simulink model "RobotArmControl"  (R2021a)
settings: Solver=FixedStepAuto  StartTime=0.0  StopTime=inf  RelTol=1e-3  EnableMultiTasking=on
InitFcn:
  | cBase=90;
  | cShoulder=90;
  | cElbow=90;
  | cWristVer=90;
  | cWristRot=90;
  | cGripper=73;
libraries: arduinolib x8
settings Model: SILPILModeSetting=veronly  ExtModeTrigDuration=2  Creator=loris  LastModifiedBy=angelo
settings OptimizationCC: EnhancedBackFolding=on  PassReuseOutputArgsAs=Individual arguments  ZeroExternalMemoryAtStartup=off  ZeroInternalMemoryAtStartup=off  MaxStackSize=64  OptimizeBlockOrder=speed  DifferentSizesBufferReuse=on  OptimizationCustomize=off  EfficientTunableParamExpr=on
settings DebuggingCC: ParameterTunabilityLossMsg=error
settings HardwareCC: ProdBitPerInt=16  ProdBitPerPointer=16  ProdBitPerSizeT=16  ProdBitPerPtrDiffT=16  ProdLargestAtomicFloat=None  ProdWordSize=8  ProdHWDeviceType=Atmel->AVR
settings SFSimCC: MATLABDynamicMemAlloc=off
settings RTWCC: SystemTargetFile=ert.tlc  HardwareBoard=Arduino Mega 2560  TemplateMakefile=ert_default_tmf  Toolchain=Arduino AVR  BuildConfiguration=Faster Runs
settings CodeAppCC: ForceParamTrailComments=on  IgnoreCustomStorageClasses=off  OperatorAnnotations=on  SimulinkDataObjDesc=on  SFDataObjDesc=on  InsertBlockDesc=on
settings ERTTargetCC: TargetLangStandard=C99 (ISO)  SupportContinuousTime=on  SupportVariableSizeSignals=on  ExtModeStaticAllocSize=2048  RootIOFormat=Structure reference

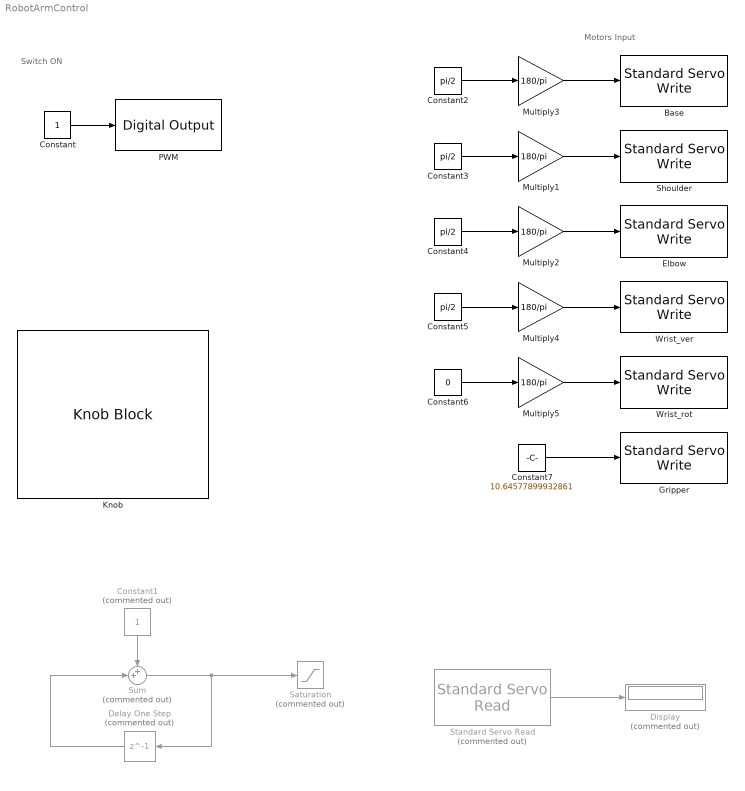
== system RobotArmControl ==
  note: Switch ON
  note: Motors Input
  Base : arduinolib/Standard Servo Write  pinNumber=11  ServoIndex=0  blockPlatform=ARDUINO
  Constant : Constant
  Constant1 : Constant  Commented=on
  Constant{2..5} (4 alike) : Constant  Value=pi/2
  Constant6 : Constant  Value=0
  Constant7 : Constant  Value=10.64577899932861
  Delay One Step : Delay  Commented=on  DelayLength=1
  Display : Display  Commented=on
  Elbow : arduinolib/Standard Servo Write  pinNumber=9  ServoIndex=1  blockPlatform=ARDUINO
  Gripper : arduinolib/Standard Servo Write  pinNumber=3  ServoIndex=2  blockPlatform=ARDUINO
  Knob : KnobBlock  ScaleMin=10  ScaleMax=73
  Multiply{1..5} (5 alike) : Gain  Gain=180/pi
  PWM : arduinolib/Digital Output  pinNumber=12  Direction=output  blockPlatform=arduino
  Saturation : Saturate  Commented=on  UpperLimit=73  LowerLimit=10
  Shoulder : arduinolib/Standard Servo Write  pinNumber=10  ServoIndex=3  blockPlatform=ARDUINO
  Standard Servo Read : arduinolib/Standard Servo Read  Commented=on  pinNumber=2  SampleTime=0.1  ServoIndex=0  blockPlatform=ARDUINO
      settings: SourceProductBaseCode=ARDUINO
  Sum : Sum  Commented=on  Inputs=++|
  Wrist_rot : arduinolib/Standard Servo Write  pinNumber=5  ServoIndex=4  blockPlatform=ARDUINO
  Wrist_ver : arduinolib/Standard Servo Write  pinNumber=6  ServoIndex=5  blockPlatform=ARDUINO
  wires:
  Constant/1 -> PWM/1
  Standard Servo Read/1 -> Display/1
  Sum/1 -> Saturation/1, Delay One Step/1
  Constant1/1 -> Sum/1
  Delay One Step/1 -> Sum/2
  Multiply3/1 -> Base/1
  Constant2/1 -> Multiply3/1
  Constant3/1 -> Multiply1/1
  Multiply1/1 -> Shoulder/1
  Multiply2/1 -> Elbow/1
  Constant4/1 -> Multiply2/1
  Constant5/1 -> Multiply4/1
  Constant6/1 -> Multiply5/1
  Multiply5/1 -> Wrist_rot/1
  Multiply4/1 -> Wrist_ver/1
  Constant7/1 -> Gripper/1
